simulink library "csu_htv_homography_to_velocity_lib"  (R2014b)
settings: Solver=ode45  StartTime=0.0  StopTime=10.0  RelTol=1e-3
undefined symbols (not defined in the file or in its folder): cam_intrinsic_matrix_c, cam_intrinsic_matrix_c_inv
libraries: util_quat_lib x4, simulink x3, util_common_lib x2, util_info_lib x1
settings Model: Creator=escrane  LastModifiedBy=mstewart

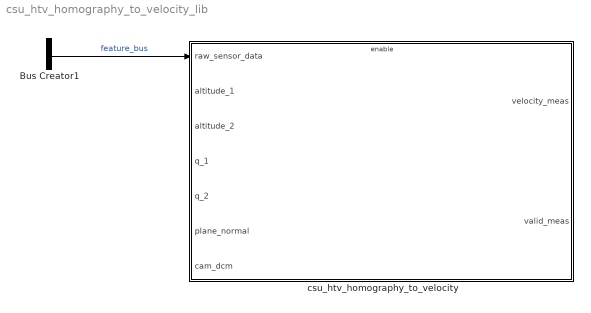
== system csu_htv_homography_to_velocity_lib ==
  Bus Creator1 : BusCreator  Inputs=2  OutDataTypeStr=Bus: feature_msg  NonVirtualBus=on
  csu_htv_homography_to_velocity : Subsystem  TreatAsAtomicUnit=on
  wires:
  ? -> Bus Creator1/2  "pixels_2"
  ? -> Bus Creator1/1  "pixels_1"
  Bus Creator1/1 -> csu_htv_homography_to_velocity/1(raw_sensor_data)  "feature_bus"

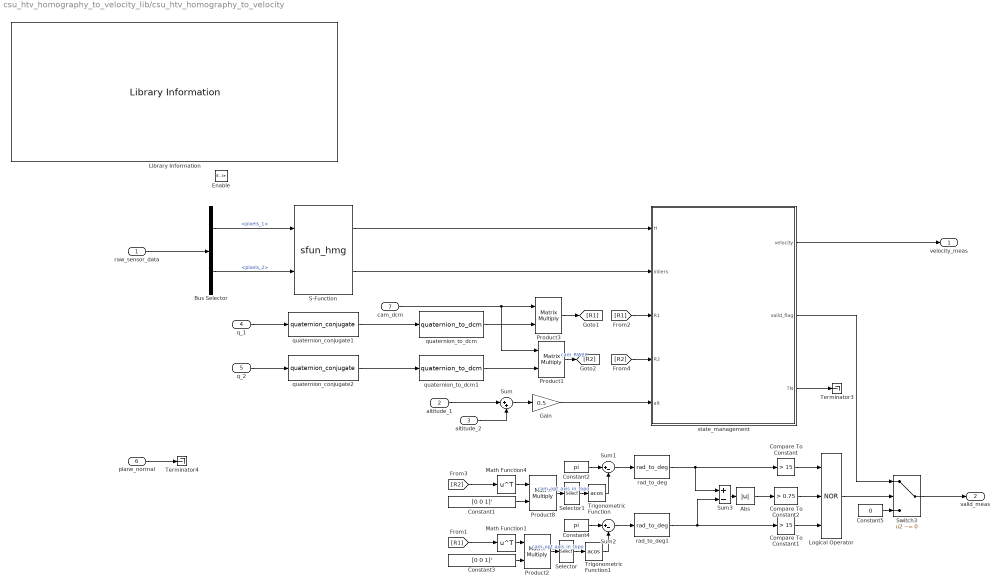
== system csu_htv_homography_to_velocity_lib/csu_htv_homography_to_velocity ==
  raw_sensor_data : Inport
  altitude_1 : Inport  Port=2
  altitude_2 : Inport  Port=3
  q_1 : Inport  Port=4
  q_2 : Inport  Port=5
  plane_normal : Inport  Port=6
  cam_dcm : Inport  Port=7
  Enable : EnablePort
  Abs : Abs
  Bus Selector : BusSelector  OutputSignals=pixels_1,pixels_2
  Compare To Constant : simulink/Logic and Bit Operations/Compare To Constant  relop=>  const=15  OutDataTypeStr=boolean
  Compare To Constant1 : simulink/Logic and Bit Operations/Compare To Constant  relop=>  const=15  OutDataTypeStr=boolean
  Compare To Constant2 : simulink/Logic and Bit Operations/Compare To Constant  relop=>  const=0.75  OutDataTypeStr=boolean
  Constant1 : Constant  Value=[0 0 1]'  VectorParams1D=off
  Constant2 : Constant  Value=pi  VectorParams1D=off
  Constant3 : Constant  Value=[0 0 1]'  VectorParams1D=off
  Constant4 : Constant  Value=pi  VectorParams1D=off
  Constant5 : Constant  Value=0  VectorParams1D=off
  Gain : Gain  Gain=0.5
  Library Information : util_info_lib/Library Information  owner='NONE'
  Logical Operator : Logic  Operator=NOR  Inputs=3  AllPortsSameDT=off  OutDataTypeStr=boolean
  Math Function1 : Math  Operator=transpose  SaturateOnIntegerOverflow=on
  Math Function4 : Math  Operator=transpose  SaturateOnIntegerOverflow=on
  Product{1..3,8} (4 alike) : Product  Multiplication=Matrix(*)  RndMeth=Zero
  S-Function : S-Function  FunctionName=sfun_hmg  Parameters=2  EnableBusSupport=off
  Selector : Selector  InputPortWidth=3  Indices=[3]
  Selector1 : Selector  InputPortWidth=3  Indices=[3]
  Sum : Sum  Inputs=|++
  Sum1 : Sum  Inputs=|+-
  Sum2 : Sum  Inputs=|+-
  Sum3 : Sum  Inputs=+-
  Switch3 : Switch  Criteria=u2 ~= 0
  Terminator3 : Terminator
  Terminator4 : Terminator
  Trigonometric Function : Trigonometry  Operator=acos
  Trigonometric Function1 : Trigonometry  Operator=acos
  quaternion_conjugate1 : util_quat_lib/quaternion_conjugate  SystemSampleTime=-1
  quaternion_conjugate2 : util_quat_lib/quaternion_conjugate  SystemSampleTime=-1
  quaternion_to_dcm : util_quat_lib/quaternion_to_dcm  SystemSampleTime=-1
  quaternion_to_dcm1 : util_quat_lib/quaternion_to_dcm  SystemSampleTime=-1
  rad_to_deg : util_common_lib/rad_to_deg  SystemSampleTime=-1
  rad_to_deg1 : util_common_lib/rad_to_deg  SystemSampleTime=-1
  state_management : MATLAB Function  TreatAsAtomicUnit=on
  velocity_meas : Outport
  valid_meas : Outport  Port=2
  wires:
  quaternion_conjugate2/1 -> quaternion_to_dcm1/1
  quaternion_conjugate1/1 -> quaternion_to_dcm/1
  Switch3/1 -> valid_meas/1
  quaternion_to_dcm1/1 -> Product1/2
  quaternion_to_dcm/1 -> Product3/2
  q_2/1 -> quaternion_conjugate2/1
  q_1/1 -> quaternion_conjugate1/1
  Product1/1 -> [R2]  "cam_RW2C"
  [R2] -> state_management/4(R2)
  [R2] -> Math Function4/1
  [R1] -> Math Function1/1
  [R1] -> state_management/3(R1)
  state_management/2(valid_flag) -> Switch3/1
  Constant5/1 -> Switch3/3
  Selector1/1 -> Trigonometric Function/1
  Product8/1 -> Selector1/1  "cam_opt_axis_in_topo"
  Selector/1 -> Trigonometric Function1/1
  Logical Operator/1 -> Switch3/2
  Compare To Constant2/1 -> Logical Operator/2
  Abs/1 -> Compare To Constant2/1
  Compare To Constant1/1 -> Logical Operator/3
  Sum3/1 -> Abs/1
  Compare To Constant/1 -> Logical Operator/1
  rad_to_deg1/1 -> Compare To Constant1/1, Sum3/2
  rad_to_deg/1 -> Sum3/1, Compare To Constant/1
  Sum2/1 -> rad_to_deg1/1
  Trigonometric Function1/1 -> Sum2/2
  Constant4/1 -> Sum2/1
  Product2/1 -> Selector/1  "cam_opt_axis_in_topo"
  Constant3/1 -> Product2/2
  Math Function1/1 -> Product2/1
  Sum1/1 -> rad_to_deg/1
  Trigonometric Function/1 -> Sum1/2
  Constant2/1 -> Sum1/1
  Constant1/1 -> Product8/2
  Math Function4/1 -> Product8/1
  plane_normal/1 -> Terminator4/1
  cam_dcm/1 -> Product1/1, Product3/1
  state_management/3(TN) -> Terminator3/1
  S-Function/2 -> state_management/2(inliers)
  Product3/1 -> [R1]
  state_management/1(velocity) -> velocity_meas/1
  S-Function/1 -> state_management/1(H)
  Bus Selector/2 -> S-Function/2  "<pixels_2>"
  Bus Selector/1 -> S-Function/1  "<pixels_1>"
  Sum/1 -> Gain/1
  altitude_2/1 -> Sum/2
  altitude_1/1 -> Sum/1
  Gain/1 -> state_management/5(alt)
  raw_sensor_data/1 -> Bus Selector/1

== matlab function csu_htv_homography_to_velocity_lib/csu_htv_homography_to_velocity/state_management ==
  data: H input; inliers input; velocity output; R1 input; R2 input; alt input; valid_flag output; cam_intrinsic_matrix_c parameter; cam_intrinsic_matrix_c_inv parameter; TN output
function [velocity, valid_flag, TN]  = conte_method(H, inliers, R1, R2, alt, cam_intrinsic_matrix_c,cam_intrinsic_matrix_c_inv)
%#codegen

% RW2C1 = cam_cam_lander_dcm *  R1 ;
% RW2C2 = cam_cam_lander_dcm *  R2 ;
RW2C1 =  R1 ;
RW2C2 =   R2 ;

TN = alt*(RW2C2'*cam_intrinsic_matrix_c_inv*H*cam_intrinsic_matrix_c*RW2C1-eye(3));

% back out T from TN
% tx = mean( TN(1,:) ./ plane_normal' );
% ty = mean( TN(2,:) ./ plane_normal' );
% tz = mean( TN(3,:) ./ plane_normal' );

tx = TN(1,3);
ty = TN(2,3);
%tz = TN(3,3);


velocity = [ tx ty ] / 0.1;
valid_flag = (sum(inliers) > 6) && ~(all(all(H==0)));
